simulink model "NeuromuscularModel_3R60_2D"  (R2019b)
settings: Solver=ode15s  StartTime=0.0  StopTime=30  MaxStep=.01  RelTol=1e-4  AbsTol=1e-6  EnableMultiTasking=on
values from neighbouring files (symbols this model uses):
  dt_visual = 1/50    (= 0.02)    [evaluateCost.m]    (also in optimize.m = 0.0333333333333)
  initialTargetAngle = 70*pi/180    (= 1.2217304764)    [setInit.m]
  LongDelay = 0.020    (= 0.02)    [ControlParams.m]
  LPreStimBFSHst = Gains(51)    [assignGains.m]
  LPreStimGASst = Gains(52)    [assignGains.m]
  LPreStimGLUst = Gains(47)    [assignGains.m]
  LPreStimHAMst = Gains(48)    [assignGains.m]
  LPreStimHFLst = Gains(46)    [assignGains.m]
  LPreStimRFst = Gains(49)    [assignGains.m]
  LPreStimSOLst = Gains(53)    [assignGains.m]
  LPreStimTAst = Gains(54)    [assignGains.m]
  LPreStimVASst = Gains(50)    [assignGains.m]
  MidDelay = 0.010    (= 0.01)    [ControlParams.m]
  RPreStimGLUsw = Gains(95)    [assignGains.m]
  RPreStimHAMsw = Gains(96)    [assignGains.m]
  RPreStimHFLsw = Gains(94)    [assignGains.m]
  RPreStimRFsw = Gains(97)    [assignGains.m]
  ShortDelay = 0.005    [ControlParams.m]
  termination_height = 0.5    [ControlParams.m]
  vy0 = paramIC(10)*.2    [setInit.m]
undefined symbols (not defined in the file or in its folder): g, hatLeftHipToCenterDistWidth, hatLeftHipToCG, initialTargetAngleR, LongLoopDelay, LPreStimHABst, LPreStimHADst, magnitude, obstacle_depth, obstacle_height, obstacle_width, obstacle_x, RPreStimHABsw, RPreStimHADsw, thetaHATref, X, Y, y0, Z
libraries: NeuroMuscularLibrary x100, sm_lib x24, nesl_utility x16, simulink x5
(part 4 of 4)

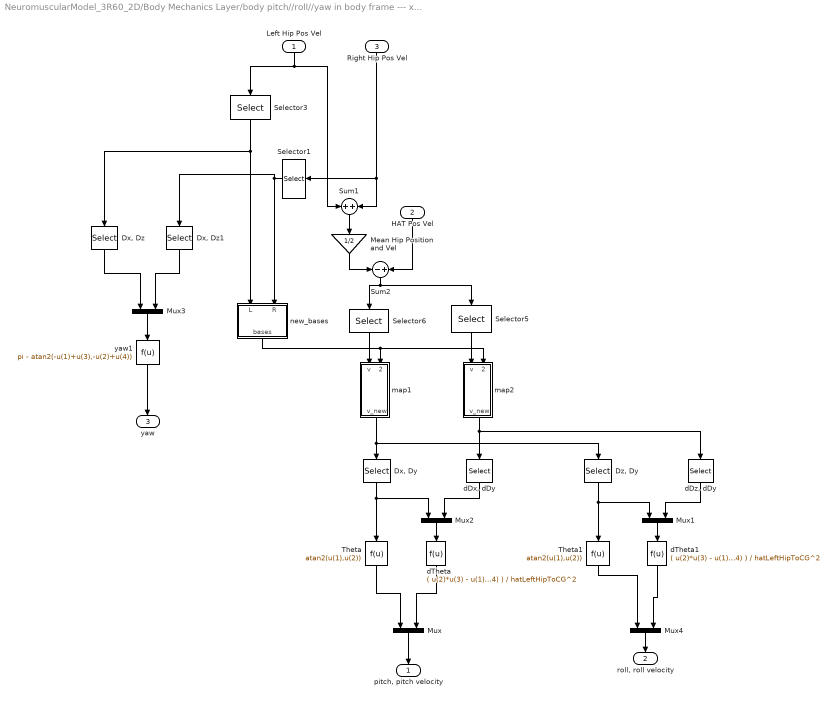
== system NeuromuscularModel_3R60_2D/Body Mechanics Layer/body pitch//roll//yaw in body frame --- x-axis: forward y-axis: leftward z-axis: parallel to gravity ==
  Left Hip Pos Vel : Inport
  HAT Pos Vel : Inport  Port=2
  Right Hip Pos Vel : Inport  Port=3
  "Dx, Dy" : Selector  InputPortWidth=3  IndexOptions=Index vector (dialog)  Indices=[1 2]  OutputSizes=1
  "Dx, Dz" : Selector  InputPortWidth=3  IndexOptions=Index vector (dialog)  Indices=[1 2]  OutputSizes=1
  "Dx, Dz1" : Selector  InputPortWidth=3  IndexOptions=Index vector (dialog)  Indices=[1 2]  OutputSizes=1
  "Dz, Dy" : Selector  InputPortWidth=3  IndexOptions=Index vector (dialog)  Indices=[3 2]  OutputSizes=1
  Mean Hip Position and Vel : Gain  Gain=1/2
  Mux{,1..4} (5 alike) : Mux  Inputs=2
  Selector1 : Selector  InputPortWidth=6  IndexOptions=Index vector (dialog)  Indices=[1 2 3]  OutputSizes=1
  Selector3 : Selector  InputPortWidth=6  IndexOptions=Index vector (dialog)  Indices=[1 2 3]  OutputSizes=1
  Selector5 : Selector  InputPortWidth=6  IndexOptions=Index vector (dialog)  Indices=[4 5 6]  OutputSizes=1
  Selector6 : Selector  InputPortWidth=6  IndexOptions=Index vector (dialog)  Indices=[1 2 3]  OutputSizes=1
  Sum1 : Sum
  Sum2 : Sum  Inputs=-+
  Theta : Fcn  Expr=atan2(u(1),u(2))
  Theta1 : Fcn  Expr=atan2(u(1),u(2))
  "dDx, dDy" : Selector  InputPortWidth=3  IndexOptions=Index vector (dialog)  Indices=[1 2]  OutputSizes=1
  "dDz, dDy" : Selector  InputPortWidth=3  IndexOptions=Index vector (dialog)  Indices=[3 2]  OutputSizes=1
  dTheta : Fcn  Expr=( u(2)*u(3) - u(1)*u(4) ) / hatLeftHipToCG^2
  dTheta1 : Fcn  Expr=( u(2)*u(3) - u(1)*u(4) ) / hatLeftHipToCG^2
  map1 : Subsystem
  map2 : Subsystem
  new_bases : Subsystem
  yaw1 : Fcn  Expr=pi - atan2(-u(1)+u(3),-u(2)+u(4))
  "pitch, pitch velocity" : Outport
  "roll, roll velocity" : Outport  Port=2
  yaw : Outport  Port=3
  wires:
  "dDx, dDy"/1 -> Mux2/2
  Mux2/1 -> dTheta/1
  HAT Pos Vel/1 -> Sum2/2
  "Dx, Dy"/1 -> Mux2/1, Theta/1
  Selector3/1 -> "Dx, Dz"/1, new_bases/1(L)
  Selector1/1 -> "Dx, Dz1"/1, new_bases/2(R)
  Theta/1 -> Mux/1
  dTheta/1 -> Mux/2
  Selector6/1 -> map1/1(v)
  map1/1(v_new) -> "Dx, Dy"/1, "Dz, Dy"/1
  new_bases/1(bases) -> map1/2(basis), map2/2(basis)
  Selector5/1 -> map2/1(v)
  map2/1(v_new) -> "dDx, dDy"/1, "dDz, dDy"/1
  "dDz, dDy"/1 -> Mux1/2
  Mux1/1 -> dTheta1/1
  "Dz, Dy"/1 -> Mux1/1, Theta1/1
  Theta1/1 -> Mux4/1
  dTheta1/1 -> Mux4/2
  "Dx, Dz"/1 -> Mux3/1
  "Dx, Dz1"/1 -> Mux3/2
  Mux3/1 -> yaw1/1
  yaw1/1 -> yaw/1
  Left Hip Pos Vel/1 -> Sum1/1, Selector3/1
  Mean Hip Position and Vel/1 -> Sum2/1
  Sum1/1 -> Mean Hip Position and Vel/1
  Sum2/1 -> Selector6/1, Selector5/1
  Mux/1 -> "pitch, pitch velocity"/1
  Mux4/1 -> "roll, roll velocity"/1
  Right Hip Pos Vel/1 -> Sum1/2, Selector1/1

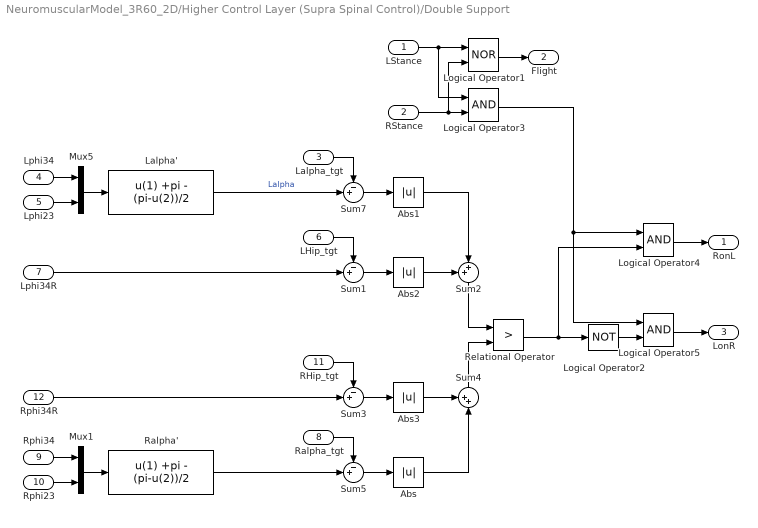
== system NeuromuscularModel_3R60_2D/Higher Control Layer (Supra Spinal Control)/Double Support ==
  LStance : Inport
  RStance : Inport  Port=2
  Lalpha_tgt : Inport  Port=3
  Lphi34 : Inport  Port=4
  Lphi23 : Inport  Port=5
  LHip_tgt : Inport  Port=6
  Lphi34R : Inport  Port=7
  Ralpha_tgt : Inport  Port=8
  Rphi34 : Inport  Port=9
  Rphi23 : Inport  Port=10
  RHip_tgt : Inport  Port=11
  Rphi34R : Inport  Port=12
  Abs{,1..3} (4 alike) : Abs  ZeroCross=off
  Lalpha' : Fcn  Expr=u(1) +pi - (pi-u(2))/2
  Logical Operator1 : Logic  Operator=NOR  AllPortsSameDT=off  OutDataTypeStr=boolean
  Logical Operator2 : Logic  Operator=NOT  AllPortsSameDT=off
  Logical Operator3 : Logic  AllPortsSameDT=off
  Logical Operator4 : Logic  AllPortsSameDT=off
  Logical Operator5 : Logic  AllPortsSameDT=off
  Mux1 : Mux  Inputs=2
  Mux5 : Mux  Inputs=2
  Ralpha' : Fcn  Expr=u(1) +pi - (pi-u(2))/2
  Relational Operator : RelationalOperator  Operator=>  ZeroCross=off  RndMeth=Nearest
  Sum{1,3,5,7} (4 alike) : Sum  Inputs=-+|
  Sum2 : Sum  Inputs=++|
  Sum4 : Sum  Inputs=++|
  RonL : Outport
  Flight : Outport  Port=2
  LonR : Outport  Port=3
  wires:
  Lalpha'/1 -> Sum7/2  "Lalpha"
  Mux5/1 -> Lalpha'/1
  Ralpha'/1 -> Sum5/2
  Mux1/1 -> Ralpha'/1
  Sum5/1 -> Abs/1
  Sum7/1 -> Abs1/1
  LStance/1 -> Logical Operator3/1, Logical Operator1/1
  RStance/1 -> Logical Operator3/2, Logical Operator1/2
  Lalpha_tgt/1 -> Sum7/1
  Lphi34/1 -> Mux5/1
  Lphi23/1 -> Mux5/2
  Ralpha_tgt/1 -> Sum5/1
  Rphi34/1 -> Mux1/1
  Rphi23/1 -> Mux1/2
  Logical Operator1/1 -> Flight/1
  LHip_tgt/1 -> Sum1/1
  Lphi34R/1 -> Sum1/2
  Sum1/1 -> Abs2/1
  Abs2/1 -> Sum2/1
  Abs1/1 -> Sum2/2
  Sum2/1 -> Relational Operator/1
  RHip_tgt/1 -> Sum3/1
  Rphi34R/1 -> Sum3/2
  Sum3/1 -> Abs3/1
  Abs/1 -> Sum4/2
  Abs3/1 -> Sum4/1
  Sum4/1 -> Relational Operator/2
  Logical Operator4/1 -> RonL/1
  Logical Operator2/1 -> Logical Operator5/2
  Logical Operator5/1 -> LonR/1
  Relational Operator/1 -> Logical Operator2/1, Logical Operator4/2
  Logical Operator3/1 -> Logical Operator5/1, Logical Operator4/1

== system NeuromuscularModel_3R60_2D/Body Mechanics Layer/body pitch//roll//yaw in body frame --- x-axis: forward y-axis: leftward z-axis: parallel to gravity/map1 ==
  v : Inport
  basis : Inport  Port=2
  Demux : Demux  Outputs=3
  Dot Product : DotProduct  InputSameDT=on  OutDataTypeStr=Inherit: Inherit via internal rule
  Dot Product1 : DotProduct  InputSameDT=on  OutDataTypeStr=Inherit: Inherit via internal rule
  Dot Product2 : DotProduct  InputSameDT=on  OutDataTypeStr=Inherit: Inherit via internal rule
  Mux3 : Mux  Inputs=3
  v_new : Outport
  wires:
  v/1 -> Dot Product2/2, Dot Product1/2, Dot Product/2
  Dot Product/1 -> Mux3/1
  Dot Product1/1 -> Mux3/2
  Dot Product2/1 -> Mux3/3
  Mux3/1 -> v_new/1  "v1"
  basis/1 -> Demux/1
  Demux/1 -> Dot Product/1
  Demux/2 -> Dot Product1/1
  Demux/3 -> Dot Product2/1

== system NeuromuscularModel_3R60_2D/Body Mechanics Layer/body pitch//roll//yaw in body frame --- x-axis: forward y-axis: leftward z-axis: parallel to gravity/map2 ==
  v : Inport
  basis : Inport  Port=2
  Demux : Demux  Outputs=3
  Dot Product : DotProduct  InputSameDT=on  OutDataTypeStr=Inherit: Inherit via internal rule
  Dot Product1 : DotProduct  InputSameDT=on  OutDataTypeStr=Inherit: Inherit via internal rule
  Dot Product2 : DotProduct  InputSameDT=on  OutDataTypeStr=Inherit: Inherit via internal rule
  Mux3 : Mux  Inputs=3
  v_new : Outport
  wires:
  v/1 -> Dot Product2/2, Dot Product1/2, Dot Product/2
  Dot Product/1 -> Mux3/1
  Dot Product1/1 -> Mux3/2
  Dot Product2/1 -> Mux3/3
  Mux3/1 -> v_new/1  "v1"
  basis/1 -> Demux/1
  Demux/1 -> Dot Product/1
  Demux/2 -> Dot Product1/1
  Demux/3 -> Dot Product2/1

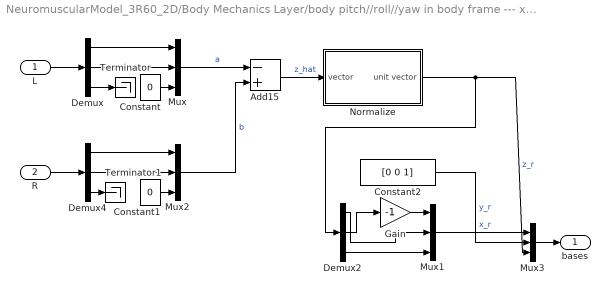
== system NeuromuscularModel_3R60_2D/Body Mechanics Layer/body pitch//roll//yaw in body frame --- x-axis: forward y-axis: leftward z-axis: parallel to gravity/new_bases ==
  L : Inport
  R : Inport  Port=2
  Add15 : Sum  Inputs=-+
  Constant : Constant  Value=0
  Constant1 : Constant  Value=0
  Constant2 : Constant  Value=[0 0 1]
  Demux : Demux  Outputs=3
  Demux2 : Demux  Outputs=3
  Demux4 : Demux  Outputs=3
  Gain : Gain  Gain=-1
  Mux{,1..3} (4 alike) : Mux  Inputs=3
  Normalize : Subsystem
  Terminator : Terminator
  Terminator1 : Terminator
  bases : Outport
  wires:
  Constant2/1 -> Mux3/2  "y_r"
  Demux2/1 -> Mux1/2
  Demux2/3 -> Mux1/3
  Demux2/2 -> Gain/1
  Add15/1 -> Normalize/1(vector)  "z_hat"
  Normalize/1(unit vector) -> Demux2/1, Mux3/3  "z_r"
  Mux2/1 -> Add15/2  "b"
  Demux4/2 -> Mux2/2
  Constant1/1 -> Mux2/3
  Demux4/3 -> Terminator1/1
  Demux4/1 -> Mux2/1
  Mux/1 -> Add15/1  "a"
  Demux/2 -> Mux/2
  Constant/1 -> Mux/3
  Demux/3 -> Terminator/1
  Demux/1 -> Mux/1
  L/1 -> Demux/1
  R/1 -> Demux4/1
  Mux3/1 -> bases/1
  Gain/1 -> Mux1/1
  Mux1/1 -> Mux3/1  "x_r"

== system NeuromuscularModel_3R60_2D/Body Mechanics Layer/body pitch//roll//yaw in body frame --- x-axis: forward y-axis: leftward z-axis: parallel to gravity/new_bases/Normalize ==
  vector : Inport
  Constant1 : Constant  Value=.5
  Math Function : Math  Operator=magnitude^2  SaturateOnIntegerOverflow=on
  Product : Product  Inputs=*/  RndMeth=Zero
  Sqrt : Math  Operator=pow  OutputSignalType=real  SaturateOnIntegerOverflow=on
  Sum of Elements : Sum  Inputs=+
  unit vector : Outport
  wires:
  Sqrt/1 -> Product/2
  Sum of Elements/1 -> Sqrt/1
  Math Function/1 -> Sum of Elements/1
  vector/1 -> Product/1, Math Function/1
  Product/1 -> unit vector/1  "x_r"
  Constant1/1 -> Sqrt/2
